simulink model "c00014M_harness"  (R2018a)
settings: Solver=FixedStepAuto  StartTime=0.0  StopTime=300  FixedStep=0.1  RelTol=1e-3
undefined symbols (not defined in the file): A1, hmax, PriorityTank, R1, R2, sigbuilder_block
(part 24 of 24)

== stateflow chart c00014M_harness/M239/Tank3/Control/Maintenance/Chart ==
  state InitialState
    entry: LiquidIn = 0;
    LiquidOut = 0;
  state Step1
    entry: LiquidIn = 0;
    LiquidOut = 1;
  state Step2
    entry: LiquidIn = 1;
    LiquidOut = 0;
  state Step3
    entry: LiquidIn = 0;
    LiquidOut = 1;
  (default) -> InitialState
  Step3 -> InitialState : [Type~=1||LiquidLevel <=0.01]
  Step2 -> InitialState [order 1] : [Type~=1]
  Step1 -> InitialState [order 1] : [Type ~= 1]
  InitialState -> Step1 : [StartMaintenance == 1 && Type ==1]
  Step1 -> Step2 [order 2] : [LiquidLevel <=0.01]
  Step2 -> Step3 [order 2] : [LiquidLevel>=hmax*0.9]
  data: Type input; StartMaintenance input; LiquidIn output; LiquidOut output; LiquidLevel input; hmax parameter

== stateflow chart c00014M_harness/M240/Tank3/Control/Maintenance/Chart ==
  state InitialState
    entry: LiquidIn = 0;
    LiquidOut = 0;
  state Step1
    entry: LiquidIn = 0;
    LiquidOut = 1;
  state Step2
    entry: LiquidIn = 1;
    LiquidOut = 0;
  state Step3
    entry: LiquidIn = 0;
    LiquidOut = 1;
  (default) -> InitialState
  Step3 -> InitialState : [Type~=1||LiquidLevel <=0.01]
  Step2 -> InitialState [order 1] : [Type~=1]
  Step1 -> InitialState [order 1] : [Type ~= 1]
  InitialState -> Step1 : [StartMaintenance == 1 && Type ==1]
  Step1 -> Step2 [order 2] : [LiquidLevel <=0.01]
  Step2 -> Step3 [order 2] : [LiquidLevel>=hmax*0.9]
  data: Type input; StartMaintenance input; LiquidIn output; LiquidOut output; LiquidLevel input; hmax parameter

== stateflow chart c00014M_harness/M241/Tank3/Control/Maintenance/Chart ==
  state InitialState
    entry: LiquidIn = 0;
    LiquidOut = 0;
  state Step1
    entry: LiquidIn = 0;
    LiquidOut = 1;
  state Step2
    entry: LiquidIn = 1;
    LiquidOut = 0;
  state Step3
    entry: LiquidIn = 0;
    LiquidOut = 1;
  (default) -> InitialState
  Step3 -> InitialState : [Type~=1||LiquidLevel <=0.01]
  Step2 -> InitialState [order 1] : [Type~=1]
  Step1 -> InitialState [order 1] : [Type ~= 1]
  InitialState -> Step1 : [StartMaintenance == 1 && Type ==1]
  Step1 -> Step2 [order 2] : [LiquidLevel <=0.01]
  Step2 -> Step3 [order 2] : [LiquidLevel>=hmax*0.9]
  data: Type input; StartMaintenance input; LiquidIn output; LiquidOut output; LiquidLevel input; hmax parameter

== stateflow chart c00014M_harness/M242/Tank3/Control/Maintenance/Chart ==
  state InitialState
    entry: LiquidIn = 0;
    LiquidOut = 0;
  state Step1
    entry: LiquidIn = 0;
    LiquidOut = 1;
  state Step2
    entry: LiquidIn = 1;
    LiquidOut = 0;
  state Step3
    entry: LiquidIn = 0;
    LiquidOut = 1;
  (default) -> InitialState
  Step3 -> InitialState : [Type~=1||LiquidLevel <=0.01]
  Step2 -> InitialState [order 1] : [Type~=1]
  Step1 -> InitialState [order 1] : [Type ~= 1]
  InitialState -> Step1 : [StartMaintenance == 1 && Type ==1]
  Step1 -> Step2 [order 2] : [LiquidLevel <=0.01]
  Step2 -> Step3 [order 2] : [LiquidLevel>=hmax*0.9]
  data: Type input; StartMaintenance input; LiquidIn output; LiquidOut output; LiquidLevel input; hmax parameter

== stateflow chart c00014M_harness/M243/Tank3/Control/Maintenance/Chart ==
  state InitialState
    entry: LiquidIn = 0;
    LiquidOut = 0;
  state Step1
    entry: LiquidIn = 0;
    LiquidOut = 1;
  state Step2
    entry: LiquidIn = 1;
    LiquidOut = 0;
  state Step3
    entry: LiquidIn = 0;
    LiquidOut = 1;
  (default) -> InitialState
  Step3 -> InitialState : [Type~=1||LiquidLevel <=0.01]
  Step2 -> InitialState [order 1] : [Type~=1]
  Step1 -> InitialState [order 1] : [Type ~= 1]
  InitialState -> Step1 : [StartMaintenance == 1 && Type ==1]
  Step1 -> Step2 [order 2] : [LiquidLevel <=0.01]
  Step2 -> Step3 [order 2] : [LiquidLevel>=hmax*0.9]
  data: Type input; StartMaintenance input; LiquidIn output; LiquidOut output; LiquidLevel input; hmax parameter

== stateflow chart c00014M_harness/M244/Tank3/Control/Maintenance/Chart ==
  state InitialState
    entry: LiquidIn = 0;
    LiquidOut = 0;
  state Step1
    entry: LiquidIn = 0;
    LiquidOut = 1;
  state Step2
    entry: LiquidIn = 1;
    LiquidOut = 0;
  state Step3
    entry: LiquidIn = 0;
    LiquidOut = 1;
  (default) -> InitialState
  Step3 -> InitialState : [Type~=1||LiquidLevel <=0.01]
  Step2 -> InitialState [order 1] : [Type~=1]
  Step1 -> InitialState [order 1] : [Type ~= 1]
  InitialState -> Step1 : [StartMaintenance == 1 && Type ==1]
  Step1 -> Step2 [order 2] : [LiquidLevel <=0.01]
  Step2 -> Step3 [order 2] : [LiquidLevel>=hmax*0.9]
  data: Type input; StartMaintenance input; LiquidIn output; LiquidOut output; LiquidLevel input; hmax parameter

== stateflow chart c00014M_harness/M245/Tank3/Control/Maintenance/Chart ==
  state InitialState
    entry: LiquidIn = 0;
    LiquidOut = 0;
  state Step1
    entry: LiquidIn = 0;
    LiquidOut = 1;
  state Step2
    entry: LiquidIn = 1;
    LiquidOut = 0;
  state Step3
    entry: LiquidIn = 0;
    LiquidOut = 1;
  (default) -> InitialState
  Step3 -> InitialState : [Type~=1||LiquidLevel <=0.01]
  Step2 -> InitialState [order 1] : [Type~=1]
  Step1 -> InitialState [order 1] : [Type ~= 1]
  InitialState -> Step1 : [StartMaintenance == 1 && Type ==1]
  Step1 -> Step2 [order 2] : [LiquidLevel <=0.01]
  Step2 -> Step3 [order 2] : [LiquidLevel>=hmax*0.9]
  data: Type input; StartMaintenance input; LiquidIn output; LiquidOut output; LiquidLevel input; hmax parameter

== stateflow chart c00014M_harness/M246/Tank3/Control/Maintenance/Chart ==
  state InitialState
    entry: LiquidIn = 0;
    LiquidOut = 0;
  state Step1
    entry: LiquidIn = 0;
    LiquidOut = 1;
  state Step2
    entry: LiquidIn = 1;
    LiquidOut = 0;
  state Step3
    entry: LiquidIn = 0;
    LiquidOut = 1;
  (default) -> InitialState
  Step3 -> InitialState : [Type~=1||LiquidLevel <=0.01]
  Step2 -> InitialState [order 1] : [Type~=1]
  Step1 -> InitialState [order 1] : [Type ~= 1]
  InitialState -> Step1 : [StartMaintenance == 1 && Type ==1]
  Step1 -> Step2 [order 2] : [LiquidLevel <=0.01]
  Step2 -> Step3 [order 2] : [LiquidLevel>=hmax*0.9]
  data: Type input; StartMaintenance input; LiquidIn output; LiquidOut output; LiquidLevel input; hmax parameter
